simulink model "TD1"  (R2022b)
settings: Solver=VariableStepAuto  StartTime=0.0  StopTime=10.0  RelTol=1e-3
values from neighbouring files (symbols this model uses):
  A = [0 1; 1 2]    [temp.m]
  B = [0 ; 1]    [temp.m]
  C = [1 0]    [temp.m]
undefined symbols (not defined in the file or in its folder): K
settings Model: Creator=simon.dumesny  LastModifiedBy=simon.dumesny

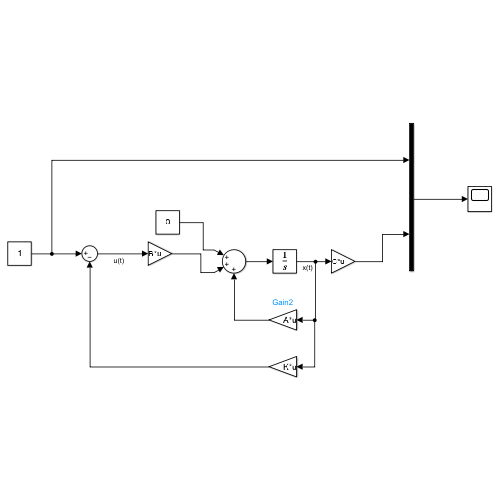
[thumbnail: Simulink's stored preview of the top-level diagram]
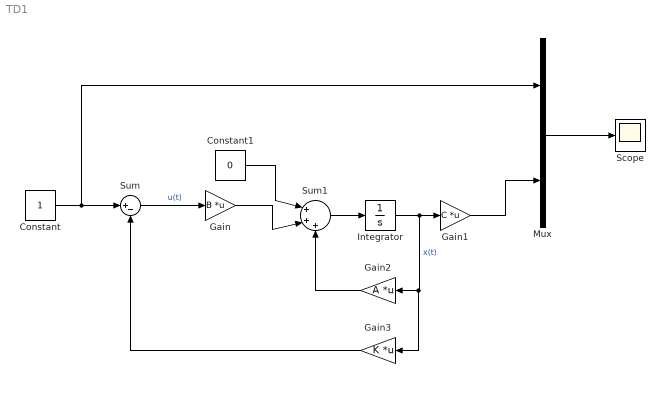
== system TD1 ==
  Constant : Constant
  Constant1 : Constant  Value=0
  Gain : Gain  Gain=B  Multiplication=Matrix(K*u)
  Gain1 : Gain  Gain=C  Multiplication=Matrix(K*u)
  Gain2 : Gain  Gain=A  Multiplication=Matrix(K*u)
  Gain3 : Gain  Gain=K  Multiplication=Matrix(K*u)
  Integrator : Integrator
  Mux : Mux  Inputs=2
  Scope : Scope
  Sum : Sum  Inputs=|+-
  Sum1 : Sum  Inputs=|+++
  wires:
  Sum/1 -> Gain/1  "u(t)"
  Gain/1 -> Sum1/2
  Sum1/1 -> Integrator/1
  Constant1/1 -> Sum1/1
  Integrator/1 -> Gain3/1, Gain2/1, Gain1/1  "x(t)"
  Gain1/1 -> Mux/2
  Mux/1 -> Scope/1
  Gain2/1 -> Sum1/3
  Gain3/1 -> Sum/2
  Constant/1 -> Mux/1, Sum/1
